simulink model "SIMULINK_NHAN_DANG"  (R2017b)
settings: Solver=FixedStepAuto  StartTime=0.0  StopTime=30  FixedStep=0.01  RelTol=1e-3
libraries: simulink x2
settings Model: Creator=DELL  LastModifiedBy=DELL

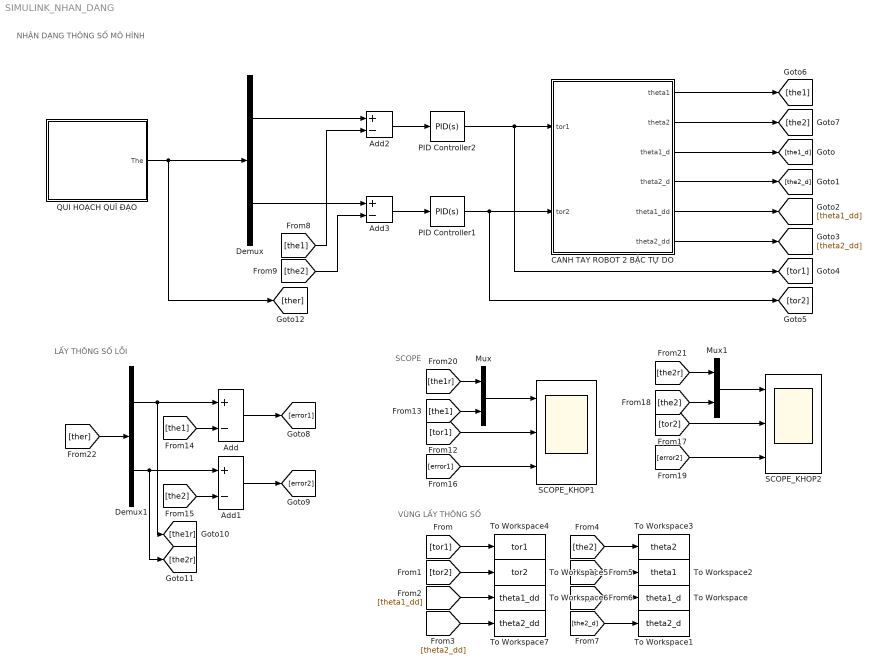
== system SIMULINK_NHAN_DANG ==
  note: LẤY THÔNG SỐ LỖI
  note: NHẬN DẠNG THÔNG SỐ MÔ HÌNH
  note: SCOPE
  note: VÙNG LẤY THÔNG SỐ
  Add{,1..3} (4 alike) : Sum  Inputs=+-
  CANH TAY ROBOT 2 BẬC TỰ DO : Subsystem
  Demux : Demux  Outputs=2
  Demux1 : Demux  Outputs=2
  Mux : Mux  Inputs=2
  Mux1 : Mux  Inputs=2
  PID Controller1 : simulink/Continuous/PID Controller  Controller=PID  TimeDomain=Continuous-time  SampleTime=-1  IntegratorMethod=Forward Euler  FilterMethod=Forward Euler  Form=Parallel  UseFilter=on  ControllerParametersSource=internal  P=30  I=16  D=5  N=100  InitialConditionSource=internal  InitialConditionForIntegrator=0  InitialConditionForFilter=0  ExternalReset=none  LimitOutput=off  UpperSaturationLimit=inf  LowerSaturationLimit=-inf  LinearizeAsGain=on  AntiWindupMode=none  Kb=1  TrackingMode=off  Kt=1  PParamMin=[]  PParamMax=[]  IParamMin=[]  IParamMax=[]  DParamMin=[]  DParamMax=[]  NParamMin=[]  NParamMax=[]  KbParamMin=[]  KbParamMax=[]  KtParamMin=[]  KtParamMax=[]  POutMin=[]  POutMax=[]  IOutMin=[]  IOutMax=[]  DOutMin=[]  DOutMax=[]  NOutMin=[]  NOutMax=[]  KbOutMin=[]  KbOutMax=[]  KtOutMin=[]  KtOutMax=[]  IntegratorOutMin=[]  IntegratorOutMax=[]  FilterOutMin=[]  FilterOutMax=[]  SumOutMin=[]  SumOutMax=[]  SumI1OutMin=[]  SumI1OutMax=[]  SumI2OutMin=[]  SumI2OutMax=[]  SumI3OutMin=[]  SumI3OutMax=[]  SumDOutMin=[]  SumDOutMax=[]  SaturationOutMin=[]  SaturationOutMax=[]  IntegratorContinuousStateAttributes=''  IntegratorStateMustResolveToSignalObject=off  IntegratorRTWStateStorageClass=Auto  FilterContinuousStateAttributes=''  FilterStateMustResolveToSignalObject=off  FilterRTWStateStorageClass=Auto  DifferentiatorICPrevScaledInput=0  DifferentiatorOutMin=[]  DifferentiatorOutMax=[]  InitialConditionSetting=State (most efficient)  FilterDiffOutCoefMin=[]  FilterDiffOutCoefMax=[]  SumDenOutMin=[]  SumDenOutMax=[]  SumNumOutMin=[]  SumNumOutMax=[]  ReciprocalOutMin=[]  ReciprocalOutMax=[]  DivideOutMin=[]  DivideOutMax=[]  TunerSelectOption=Transfer Function Based (PID Tuner App)
  PID Controller2 : simulink/Continuous/PID Controller  Controller=PID  TimeDomain=Continuous-time  SampleTime=-1  IntegratorMethod=Forward Euler  FilterMethod=Forward Euler  Form=Parallel  UseFilter=on  ControllerParametersSource=internal  P=30  I=15  D=10  N=100  InitialConditionSource=internal  InitialConditionForIntegrator=0  InitialConditionForFilter=0  ExternalReset=none  LimitOutput=off  UpperSaturationLimit=inf  LowerSaturationLimit=-inf  LinearizeAsGain=on  AntiWindupMode=none  Kb=1  TrackingMode=off  Kt=1  PParamMin=[]  PParamMax=[]  IParamMin=[]  IParamMax=[]  DParamMin=[]  DParamMax=[]  NParamMin=[]  NParamMax=[]  KbParamMin=[]  KbParamMax=[]  KtParamMin=[]  KtParamMax=[]  POutMin=[]  POutMax=[]  IOutMin=[]  IOutMax=[]  DOutMin=[]  DOutMax=[]  NOutMin=[]  NOutMax=[]  KbOutMin=[]  KbOutMax=[]  KtOutMin=[]  KtOutMax=[]  IntegratorOutMin=[]  IntegratorOutMax=[]  FilterOutMin=[]  FilterOutMax=[]  SumOutMin=[]  SumOutMax=[]  SumI1OutMin=[]  SumI1OutMax=[]  SumI2OutMin=[]  SumI2OutMax=[]  SumI3OutMin=[]  SumI3OutMax=[]  SumDOutMin=[]  SumDOutMax=[]  SaturationOutMin=[]  SaturationOutMax=[]  IntegratorContinuousStateAttributes=''  IntegratorStateMustResolveToSignalObject=off  IntegratorRTWStateStorageClass=Auto  FilterContinuousStateAttributes=''  FilterStateMustResolveToSignalObject=off  FilterRTWStateStorageClass=Auto  DifferentiatorICPrevScaledInput=0  DifferentiatorOutMin=[]  DifferentiatorOutMax=[]  InitialConditionSetting=State (most efficient)  FilterDiffOutCoefMin=[]  FilterDiffOutCoefMax=[]  SumDenOutMin=[]  SumDenOutMax=[]  SumNumOutMin=[]  SumNumOutMax=[]  ReciprocalOutMin=[]  ReciprocalOutMax=[]  DivideOutMin=[]  DivideOutMax=[]  TunerSelectOption=Transfer Function Based (PID Tuner App)
  QUI HOẠCH QUĨ ĐẠO : Subsystem
  SCOPE_KHOP1 : Scope  NumInputPorts=3
  SCOPE_KHOP2 : Scope  NumInputPorts=3
  To Workspace : ToWorkspace  VariableName=theta1_d  SaveFormat=Structure With Time  SampleTime=-1
  To Workspace1 : ToWorkspace  VariableName=theta2_d  SaveFormat=Structure With Time  SampleTime=-1
  To Workspace2 : ToWorkspace  VariableName=theta1  SaveFormat=Structure With Time  SampleTime=-1
  To Workspace3 : ToWorkspace  VariableName=theta2  SaveFormat=Structure With Time  SampleTime=-1
  To Workspace4 : ToWorkspace  VariableName=tor1  SaveFormat=Structure With Time  SampleTime=-1
  To Workspace5 : ToWorkspace  VariableName=tor2  SaveFormat=Structure With Time  SampleTime=-1
  To Workspace6 : ToWorkspace  VariableName=theta1_dd  SaveFormat=Structure With Time  SampleTime=-1
  To Workspace7 : ToWorkspace  VariableName=theta2_dd  SaveFormat=Structure With Time  SampleTime=-1
  wires:
  QUI HOẠCH QUĨ ĐẠO/1(The) -> [ther], Demux/1
  [tor1] -> To Workspace4/1
  [the2] -> To Workspace3/1
  [tor2] -> To Workspace5/1
  [theta1_dd] -> To Workspace6/1
  [theta2_dd] -> To Workspace7/1
  [the1] -> To Workspace2/1
  [the1_d] -> To Workspace/1
  [the2_d] -> To Workspace1/1
  CANH TAY ROBOT 2 BẬC TỰ DO/3(theta1_d) -> [the1_d]
  CANH TAY ROBOT 2 BẬC TỰ DO/4(theta2_d) -> [the2_d]
  CANH TAY ROBOT 2 BẬC TỰ DO/5(theta1_dd) -> [theta1_dd]
  CANH TAY ROBOT 2 BẬC TỰ DO/6(theta2_dd) -> [theta2_dd]
  CANH TAY ROBOT 2 BẬC TỰ DO/1(theta1) -> [the1]
  CANH TAY ROBOT 2 BẬC TỰ DO/2(theta2) -> [the2]
  [tor1] -> SCOPE_KHOP1/2
  Demux1/1 -> [the1r], Add/1
  Demux1/2 -> [the2r], Add1/1
  [the1] -> Add/2
  [the2] -> Add1/2
  Add/1 -> [error1]
  Add1/1 -> [error2]
  [error1] -> SCOPE_KHOP1/3
  [tor2] -> SCOPE_KHOP2/2
  [error2] -> SCOPE_KHOP2/3
  [the1] -> Mux/2
  Mux/1 -> SCOPE_KHOP1/1
  [the1r] -> Mux/1
  [the2r] -> Mux1/1
  [the2] -> Mux1/2
  Mux1/1 -> SCOPE_KHOP2/1
  [ther] -> Demux1/1
  PID Controller1/1 -> [tor2], CANH TAY ROBOT 2 BẬC TỰ DO/2(tor2)
  Demux/1 -> Add2/1
  Add2/1 -> PID Controller2/1
  PID Controller2/1 -> [tor1], CANH TAY ROBOT 2 BẬC TỰ DO/1(tor1)
  Add3/1 -> PID Controller1/1
  Demux/2 -> Add3/1
  [the1] -> Add2/2
  [the2] -> Add3/2

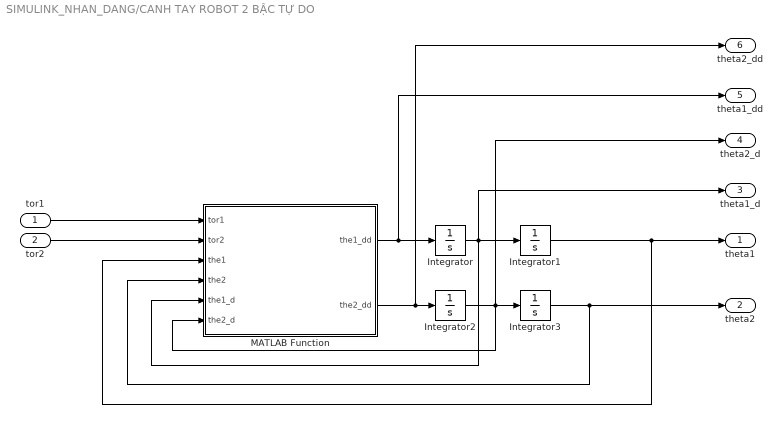
== system SIMULINK_NHAN_DANG/CANH TAY ROBOT 2 BẬC TỰ DO ==
  tor1 : Inport
  tor2 : Inport  Port=2
  Integrator{,1..3} (4 alike) : Integrator
  MATLAB Function : MATLAB Function  TreatAsAtomicUnit=on
  theta1 : Outport
  theta2 : Outport  Port=2
  theta1_d : Outport  Port=3
  theta2_d : Outport  Port=4
  theta1_dd : Outport  Port=5
  theta2_dd : Outport  Port=6
  wires:
  Integrator3/1 -> theta2/1, MATLAB Function/4(the2)
  Integrator1/1 -> theta1/1, MATLAB Function/3(the1)
  tor1/1 -> MATLAB Function/1(tor1)
  Integrator2/1 -> theta2_d/1, MATLAB Function/6(the2_d), Integrator3/1
  tor2/1 -> MATLAB Function/2(tor2)
  Integrator/1 -> theta1_d/1, MATLAB Function/5(the1_d), Integrator1/1
  MATLAB Function/2(the2_dd) -> theta2_dd/1, Integrator2/1
  MATLAB Function/1(the1_dd) -> theta1_dd/1, Integrator/1

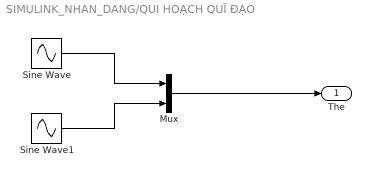
== system SIMULINK_NHAN_DANG/QUI HOẠCH QUĨ ĐẠO ==
  Mux : Mux  Inputs=2
  Sine Wave : Sin  Amplitude=pi/6  Frequency=2*pi*0.1  SampleTime=0
  Sine Wave1 : Sin  Amplitude=pi/6  Frequency=2*pi*0.1  Phase=pi/6  SampleTime=0
  The : Outport
  wires:
  Sine Wave/1 -> Mux/1
  Sine Wave1/1 -> Mux/2
  Mux/1 -> The/1

== matlab function SIMULINK_NHAN_DANG/CANH TAY ROBOT 2 BẬC TỰ DO/MATLAB Function ==
  data: the1_dd output; tor1 input; tor2 input; the1 input; the2 input; the1_d input; the2_dd output; the2_d input
function [the1_dd,the2_dd] = PTVP(tor1,tor2,the1,the2,the1_d,the2_d)
J1=0.05;
J2=0.05;
m1=1;
m2=1;
m3=0;%Khoi luong cua hai khop
l1=1;
l2=1;
lc1=0.4;
lc2=0.4;
g=9.81;
H11=J1+J2+m1*(lc1^2)+m2*((l1^2)+(lc2^2)+2*l1*lc2*cos(the2))+m3*(l1*l1+l2*l2+2*l1*l2*cos(the2));
H22=J2+m2*lc2*lc2+m3*l2*l2;
H12=J2+m2*(lc2*lc2+l1*lc2*cos(the2))+m3*(l2*l2+2*l1*l2*cos(the2));
H21=H12;
H=[H11 H12;
   H21 H22];
h=m2*l1*lc2*sin(the2);

V=[-h*the2_d   -h*the1_d - h*the2_d;
   -h*the1_d    0];
g1=m1*lc1*g*cos(the1)+m2*g*(lc2*cos(the1+the2)+l1*cos(the1));
g2=m2*lc2*g*cos(the1+the2);
G=[g1;
    g2];
tor=[tor1;
     tor2;];
the_dd=pinv(H)*(tor-G-V*[the1_d;the2_d]);
%-diag([1;1])*[the1_d;the2_d]
the1_dd=the_dd(1);
the2_dd=the_dd(2);
end
